simulink model "MeasModelCompare_throttle"  (R2014b)
settings: Solver=ode45  StartTime=0.0  StopTime=10.0  RelTol=1e-5  AbsTol=1e-5
values from neighbouring files (symbols this model uses):
  AirStep =     [AirStep.mat]
  tau_th = 0.032    [Init_Project1.m]
settings Model: ExtModeAutoUpdateStatusClock=off  Creator=oberg  LastModifiedBy=danfa688
settings DataIOCC: SignalLoggingSaveFormat=ModelDataLogs  SignalLoggingName=sigsOut
settings OptimizationCC: ExpressionDepthLimit=2147483647
settings DebuggingCC: ConsistencyChecking=warning  SaveWithParameterizedLinksMsg=none  UnderspecifiedInitializationDetection=Classic  MergeDetectMultiDrivingBlocksExec=none  SignalResolutionControl=TryResolveAllWithWarning  SolverPrmCheckMsg=none  MultiTaskDSMMsg=warning  MultiTaskCondExecSysMsg=none  FcnCallInpInsideContextMsg=UseLocalSettings  StateNameClashWarn=warning
settings HardwareCC: TargetUnknown=on
settings RTWCC: IncludeERTFirstTime=on
settings GRTTargetCC: CombineOutputUpdateFcns=off  GRTInterface=on

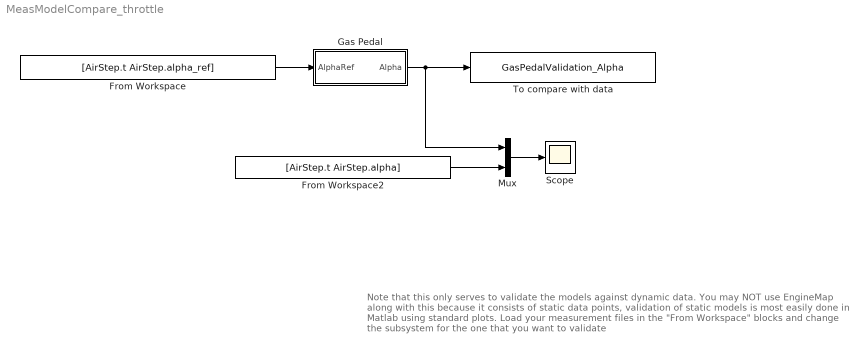
== system MeasModelCompare_throttle ==
  note: Note that this only serves to validate the models against dynamic data.
      | You may NOT use EngineMap along with this because it consists of static data points,
      | validation of static models is most easily done in Matlab using standard plots.
      |
      | Load your measurement files in the "From Workspace" blocks
      | and change the subsystem for the one that you want to validate
  From Workspace : FromWorkspace  VariableName=[AirStep.t AirStep.alpha_ref]  SampleTime=0
  From Workspace2 : FromWorkspace  VariableName=[AirStep.t AirStep.alpha]  SampleTime=0
  Gas Pedal : Subsystem
  Mux : Mux  Inputs=2
  Scope : Scope
  To compare with data : ToWorkspace  VariableName=GasPedalValidation_Alpha  SaveFormat=Structure With Time  SampleTime=-1
  wires:
  Gas Pedal/1(Alpha) -> To compare with data/1, Mux/1
  From Workspace/1 -> Gas Pedal/1(AlphaRef)
  From Workspace2/1 -> Mux/2
  Mux/1 -> Scope/1

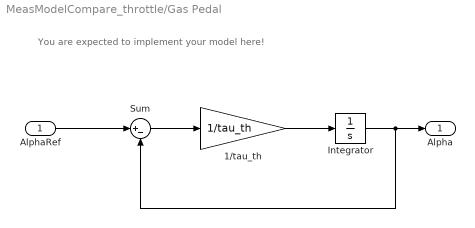
== system MeasModelCompare_throttle/Gas Pedal ==
  note: You are expected to implement your model here!
  AlphaRef : Inport
  1/tau_th : Gain  Gain=1/tau_th  SaturateOnIntegerOverflow=on  OutDataTypeStr=Inherit: Same as input  ParamDataTypeStr=Inherit: Same as input
  Integrator : Integrator  InitialCondition=AirStep.alpha_ref(1)
  Sum : Sum  Inputs=|+-  SaturateOnIntegerOverflow=on
  Alpha : Outport
  wires:
  AlphaRef/1 -> Sum/1
  Sum/1 -> 1/tau_th/1
  Integrator/1 -> Alpha/1, Sum/2
  1/tau_th/1 -> Integrator/1
